simulink model "testGrinding"  (R2025a)
settings: Solver=VariableStepAuto  StartTime=0.0  StopTime=10.0  RelTol=1e-3
libraries: StdLib x9, ProductionLinePLib x1
settings Model: Creator=peter  LastModifiedBy=peter
settings RTWCC: GPUComputeCapability=3.5

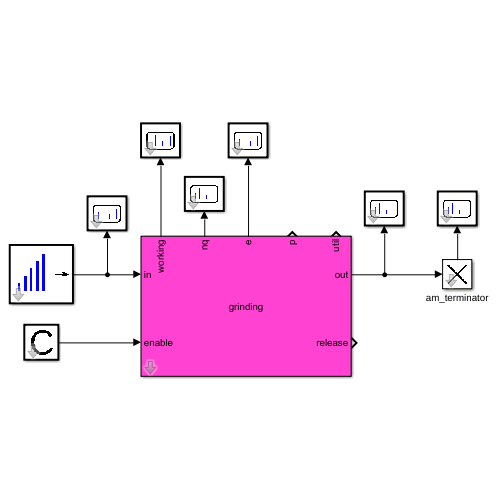
[thumbnail: Simulink's stored preview of the top-level diagram]
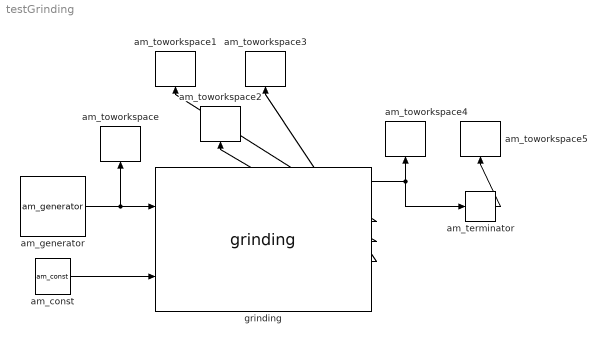
== system testGrinding ==
  am_const : StdLib/am_const  value=true  sendTime=[0,1]  debug=0
  am_generator : StdLib/am_generator  tG=300  n0=1  nG=30  tD=[0,2]  debug=0
  am_terminator : StdLib/am_terminator  tau=[0,1]  debug=0
  am_toworkspace : StdLib/am_toworkspace  varname="\"o1\""  t0=0  format="\"vector\""  tau=[0,5]  debug=0
  am_toworkspace1 : StdLib/am_toworkspace  varname="\"o2\""  t0=0  format="\"vector\""  tau=[0,5]  debug=0
  am_toworkspace2 : StdLib/am_toworkspace  varname="\"o3\""  t0=0  format="\"vector\""  tau=[0,5]  debug=0
  am_toworkspace3 : StdLib/am_toworkspace  varname="\"o4\""  t0=0  format="\"vector\""  tau=[0,5]  debug=0
  am_toworkspace4 : StdLib/am_toworkspace  varname="\"o5\""  t0=0  format="\"vector\""  tau=[0,5]  debug=0
  am_toworkspace5 : StdLib/am_toworkspace  varname="\"o6\""  t0=0  format="\"vector\""  tau=[0,5]  debug=0
  grinding : ProductionLinePLib/grinding  vfr1=0.48  vfr2=0.19  vfr3=0.03  vc=30  max_fifo=400  tauInt=[0,100]  tauCont=[0,100]  tau=[0,1]  debug=0
  wires:
  am_terminator/1 -> am_toworkspace5/1
  am_generator/1 -> am_toworkspace/1, grinding/1
  am_const/1 -> grinding/2
  grinding/1 -> am_toworkspace4/1, am_terminator/1
  grinding/3 -> am_toworkspace1/1
  grinding/4 -> am_toworkspace2/1
  grinding/5 -> am_toworkspace3/1
